simulink model "plotter_rigid_body"  (R2025a)
settings: Solver=VariableStepAuto  StartTime=0.0  StopTime=2  MaxStep=1e-3  RelTol=1e-3
values from neighbouring files (symbols this model uses):
  B_m = 0.000002    (= 2e-06)    [parameters.m]
  g = 9.8    [parameters.m]
  Gr = 1/30    (= 0.0333333333333)    [parameters.m]
  J_m = 0.000004    (= 4e-06)    [parameters.m]
  K_t = 0.009    [parameters.m]
  L = 0.3    [cinematic_sim.m]    (also in parameters.m)
  L_a = 0.0023    [parameters.m]
  m = 0.1    [parameters.m]
  R = 0.017    [parameters.m]
  R_a = 2.182    [parameters.m]
libraries: slpidlib x2
settings Model: SimulationMode=accelerator  Creator=bruno  LastModifiedBy=bruno

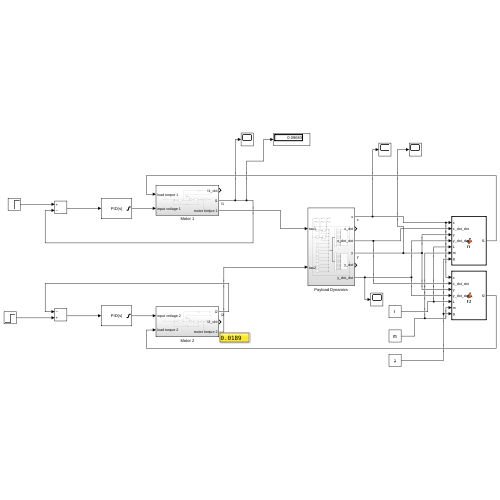
[thumbnail: Simulink's stored preview of the top-level diagram]
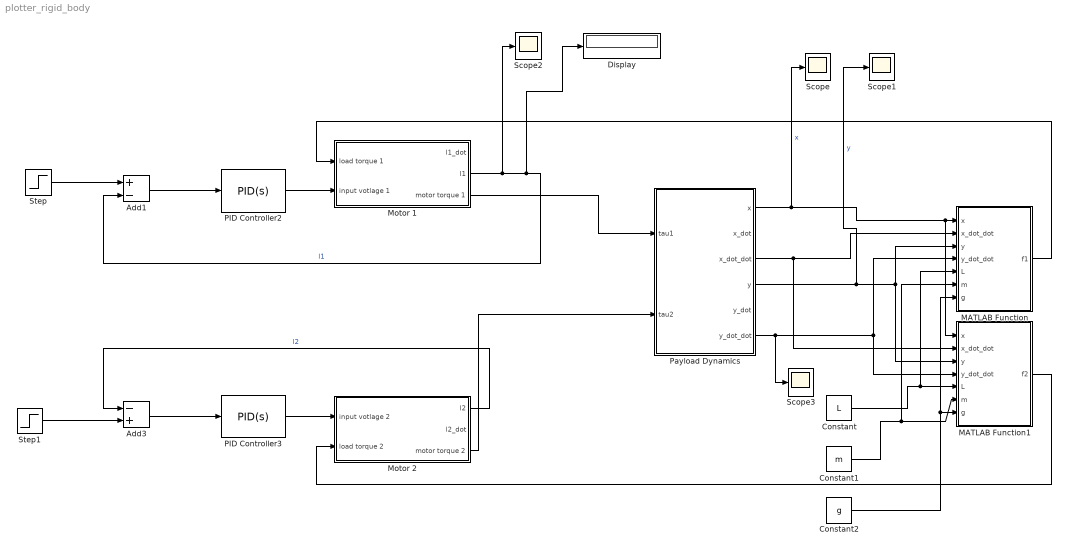
== system plotter_rigid_body ==
  Add1 : Sum  Inputs=+-
  Add3 : Sum  Inputs=-+
  Constant : Constant  Value=L
  Constant1 : Constant  Value=m
  Constant2 : Constant  Value=g
  Display : Display
  MATLAB Function : MATLAB Function  TreatAsAtomicUnit=on
  MATLAB Function1 : MATLAB Function  TreatAsAtomicUnit=on
  Motor 1 : Subsystem
  Motor 2 : Subsystem
  PID Controller2 : slpidlib/PID Controller  Controller=PID  Form=Parallel  TimeDomain=Continuous-time  UseExternalTs=off  SampleTime=-1  IntegratorMethod=Forward Euler  FilterMethod=Forward Euler  ControllerParametersSource=internal  P=7486.4932520919  I=24098.7164203864  UseKiTs=off  D=516.754104749892  UseExternalDerivativeSource=off  N=63057.2759663465  UseFilter=on  TunerSelectOption=Transfer Function Based (PID Tuner App)  InitialConditionSource=internal  InitialConditionForIntegrator=0  InitialConditionForFilter=0  DifferentiatorICPrevScaledInput=0  ExternalReset=none  TrackingMode=off  Kt=1  LimitOutput=on  SatLimitsSource=internal  UpperSaturationLimit=6  LowerSaturationLimit=-6  LinearizeAsGain=on  AntiWindupMode=none  Kb=1  LimitIntegrator=off  UpperIntegratorSaturationLimit=inf  LowerIntegratorSaturationLimit=-inf  POutMin=[]  POutMax=[]  IOutMin=[]  IOutMax=[]  DOutMin=[]  DOutMax=[]  NOutMin=[]  NOutMax=[]  SumOutMin=[]  SumOutMax=[]  SaturationOutMin=[]  SaturationOutMax=[]  PParamMin=[]  PParamMax=[]  IParamMin=[]  IParamMax=[]  DParamMin=[]  DParamMax=[]  NParamMin=[]  NParamMax=[]  KbParamMin=[]  KbParamMax=[]  KtParamMin=[]  KtParamMax=[]  KbOutMin=[]  KbOutMax=[]  KtOutMin=[]  KtOutMax=[]  IntegratorOutMin=[]  IntegratorOutMax=[]  FilterOutMin=[]  FilterOutMax=[]  SumI1OutMin=[]  SumI1OutMax=[]  SumI2OutMin=[]  SumI2OutMax=[]  SumI3OutMin=[]  SumI3OutMax=[]  SumI4OutMin=[]  SumI4OutMax=[]  SumDOutMin=[]  SumDOutMax=[]  DifferentiatorOutMin=[]  DifferentiatorOutMax=[]  FilterDiffOutCoefMin=[]  FilterDiffOutCoefMax=[]  ReciprocalOutMin=[]  ReciprocalOutMax=[]  SumDenOutMin=[]  SumDenOutMax=[]  SumNumOutMin=[]  SumNumOutMax=[]  DivideOutMin=[]  DivideOutMax=[]  UdiffTsProdOutMin=[]  UdiffTsProdOutMax=[]  NTsProdOutMin=[]  NTsProdOutMax=[]  UintegralTsProdOutMin=[]  UintegralTsProdOutMax=[]  UngainTsProdOutMin=[]  UngainTsProdOutMax=[]  ClampingZeroOutDataTypeStr=Inherit: Inherit via back propagation  ClampingZeroOutMin=[]  ClampingZeroOutMax=[]  FilterDenConstantOutDataTypeStr=Inherit: Inherit via back propagation  FilterDenConstantOutMin=[]  FilterDenConstantOutMax=[]  PCopyOutDataTypeStr=Inherit: Inherit via back propagation  PCopyOutMin=[]  PCopyOutMax=[]  NCopyOutDataTypeStr=Inherit: Inherit via back propagation  NCopyOutMin=[]  NCopyOutMax=[]  IntegratorContinuousStateAttributes=''  IntegratorStateMustResolveToSignalObject=off  IntegratorRTWStateStorageClass=Auto  FilterContinuousStateAttributes=''  FilterStateMustResolveToSignalObject=off  FilterRTWStateStorageClass=Auto  ParallelPVariant=InternalParameters  IdealPVariant=Disabled  IVariant=InternalParameters  DVariant=InternalParameters  IntegratorVariant=Continuous  SatVariant=Enabled  AWVariant=Passthrough  PCopyVariant=Disabled  TRVariant=Disabled  FdbkBlocksVariant=Forward  IdealPFdbkVariant=Disabled  SatFdbkVariant=Disabled  DerivativeFilterVariant=ContFilter  NVariant=InternalParameters  NCopyVariant=Disabled  FilterICVariant=InternalICsFilter  IntegratorICVariant=InternalICs  ExternalResetVariant=Disabled  TRSumVariant=Passthrough  SumFdbkVariant=Disabled  SumVariant=Sum_PID  TsampFilterVariant=InternalTs  TsampNgainVariant=Passthrough  TsampIntegralVariant=Disabled_SignalSpec  ExternalSaturationOutDataTypeStr=Inherit: Same as second input  DerivativeSourceVariant=ErrorSignal  PreIntVariant=InternalPreInt
  PID Controller3 : slpidlib/PID Controller  Controller=PID  Form=Parallel  TimeDomain=Continuous-time  UseExternalTs=off  SampleTime=-1  IntegratorMethod=Forward Euler  FilterMethod=Forward Euler  ControllerParametersSource=internal  P=7486.4932520919  I=24098.7164203864  UseKiTs=off  D=516.754104749892  UseExternalDerivativeSource=off  N=63057.2759663465  UseFilter=on  TunerSelectOption=Transfer Function Based (PID Tuner App)  InitialConditionSource=internal  InitialConditionForIntegrator=0  InitialConditionForFilter=0  DifferentiatorICPrevScaledInput=0  ExternalReset=none  TrackingMode=off  Kt=1  LimitOutput=on  SatLimitsSource=internal  UpperSaturationLimit=6  LowerSaturationLimit=-6  LinearizeAsGain=on  AntiWindupMode=none  Kb=1  LimitIntegrator=off  UpperIntegratorSaturationLimit=inf  LowerIntegratorSaturationLimit=-inf  POutMin=[]  POutMax=[]  IOutMin=[]  IOutMax=[]  DOutMin=[]  DOutMax=[]  NOutMin=[]  NOutMax=[]  SumOutMin=[]  SumOutMax=[]  SaturationOutMin=[]  SaturationOutMax=[]  PParamMin=[]  PParamMax=[]  IParamMin=[]  IParamMax=[]  DParamMin=[]  DParamMax=[]  NParamMin=[]  NParamMax=[]  KbParamMin=[]  KbParamMax=[]  KtParamMin=[]  KtParamMax=[]  KbOutMin=[]  KbOutMax=[]  KtOutMin=[]  KtOutMax=[]  IntegratorOutMin=[]  IntegratorOutMax=[]  FilterOutMin=[]  FilterOutMax=[]  SumI1OutMin=[]  SumI1OutMax=[]  SumI2OutMin=[]  SumI2OutMax=[]  SumI3OutMin=[]  SumI3OutMax=[]  SumI4OutMin=[]  SumI4OutMax=[]  SumDOutMin=[]  SumDOutMax=[]  DifferentiatorOutMin=[]  DifferentiatorOutMax=[]  FilterDiffOutCoefMin=[]  FilterDiffOutCoefMax=[]  ReciprocalOutMin=[]  ReciprocalOutMax=[]  SumDenOutMin=[]  SumDenOutMax=[]  SumNumOutMin=[]  SumNumOutMax=[]  DivideOutMin=[]  DivideOutMax=[]  UdiffTsProdOutMin=[]  UdiffTsProdOutMax=[]  NTsProdOutMin=[]  NTsProdOutMax=[]  UintegralTsProdOutMin=[]  UintegralTsProdOutMax=[]  UngainTsProdOutMin=[]  UngainTsProdOutMax=[]  ClampingZeroOutDataTypeStr=Inherit: Inherit via back propagation  ClampingZeroOutMin=[]  ClampingZeroOutMax=[]  FilterDenConstantOutDataTypeStr=Inherit: Inherit via back propagation  FilterDenConstantOutMin=[]  FilterDenConstantOutMax=[]  PCopyOutDataTypeStr=Inherit: Inherit via back propagation  PCopyOutMin=[]  PCopyOutMax=[]  NCopyOutDataTypeStr=Inherit: Inherit via back propagation  NCopyOutMin=[]  NCopyOutMax=[]  IntegratorContinuousStateAttributes=''  IntegratorStateMustResolveToSignalObject=off  IntegratorRTWStateStorageClass=Auto  FilterContinuousStateAttributes=''  FilterStateMustResolveToSignalObject=off  FilterRTWStateStorageClass=Auto  ParallelPVariant=InternalParameters  IdealPVariant=Disabled  IVariant=InternalParameters  DVariant=InternalParameters  IntegratorVariant=Continuous  SatVariant=Enabled  AWVariant=Passthrough  PCopyVariant=Disabled  TRVariant=Disabled  FdbkBlocksVariant=Forward  IdealPFdbkVariant=Disabled  SatFdbkVariant=Disabled  DerivativeFilterVariant=ContFilter  NVariant=InternalParameters  NCopyVariant=Disabled  FilterICVariant=InternalICsFilter  IntegratorICVariant=InternalICs  ExternalResetVariant=Disabled  TRSumVariant=Passthrough  SumFdbkVariant=Disabled  SumVariant=Sum_PID  TsampFilterVariant=InternalTs  TsampNgainVariant=Passthrough  TsampIntegralVariant=Disabled_SignalSpec  ExternalSaturationOutDataTypeStr=Inherit: Same as second input  DerivativeSourceVariant=ErrorSignal  PreIntVariant=InternalPreInt
  Payload Dynamics : Subsystem
  Scope{,1..3} (4 alike) : Scope
      Scope settings: ActiveDisplayYMinimum=0.1206169656337359  ActiveDisplayYMaximum=0.27436852673253087
      Scope1 settings: ActiveDisplayYMinimum=-0.00020832759673911072  ActiveDisplayYMaximum=0.18372931257695557
      Scope2 settings: ActiveDisplayYMinimum=-1  ActiveDisplayYMaximum=1  DataLoggingVariableName=ScopeData2
      Scope3 settings: ActiveDisplayYMinimum=-22.86647819571678  ActiveDisplayYMaximum=32.004217087156384  DataLoggingVariableName=ScopeData3
  Step : Step  Time=0  After=0.15  SampleTime=0
  Step1 : Step  Time=0  After=0.15  SampleTime=0
  wires:
  PID Controller2/1 -> Motor 1/2(input votlage 1)
  Add1/1 -> PID Controller2/1
  Step/1 -> Add1/1
  Add3/1 -> PID Controller3/1
  Step1/1 -> Add3/2
  Motor 1/2(l1) -> Scope2/1, Display/1, Add1/2  "l1"
  PID Controller3/1 -> Motor 2/1(input votlage 2)
  Motor 2/1(l2) -> Add3/1  "l2"
  Constant2/1 -> MATLAB Function1/7(g), MATLAB Function/7(g)
  Motor 2/3(motor torque 2) -> Payload Dynamics/2(tau2)
  Motor 1/3(motor torque 1) -> Payload Dynamics/1(tau1)
  Payload Dynamics/1(x) -> Scope/1, MATLAB Function1/1(x), MATLAB Function/1(x)  "x"
  Payload Dynamics/3(x_dot_dot) -> MATLAB Function1/2(x_dot_dot), MATLAB Function/2(x_dot_dot)
  Payload Dynamics/4(y) -> Scope1/1, MATLAB Function1/3(y), MATLAB Function/3(y)  "y"
  Payload Dynamics/6(y_dot_dot) -> Scope3/1, MATLAB Function1/4(y_dot_dot), MATLAB Function/4(y_dot_dot)
  Constant/1 -> MATLAB Function1/5(L), MATLAB Function/5(L)
  Constant1/1 -> MATLAB Function/6(m), MATLAB Function1/6(m)
  MATLAB Function/1(f1) -> Motor 1/1(load torque 1)
  MATLAB Function1/1(f2) -> Motor 2/2(load torque 2)

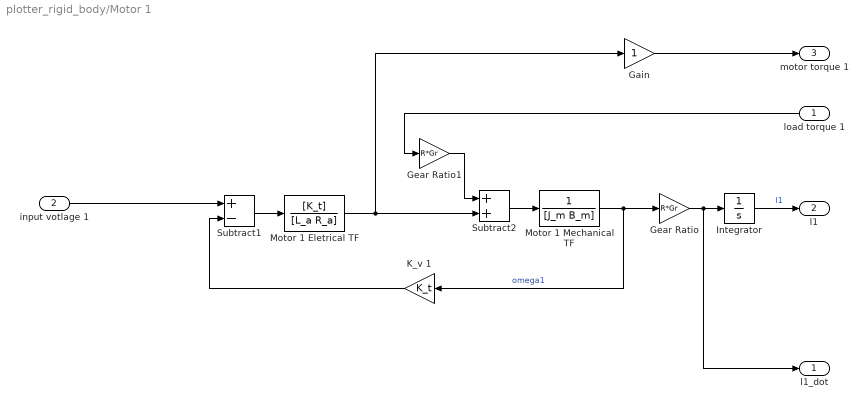
== system plotter_rigid_body/Motor 1 ==
  load torque 1 : Inport
  input votlage 1 : Inport  Port=2
  Gain : Gain
  Gear Ratio : Gain  Gain=R*Gr
  Gear Ratio1 : Gain  Gain=R*Gr
  Integrator : Integrator  InitialCondition=0.25
  K_v 1 : Gain  Gain=K_t
  Motor 1 Eletrical TF : TransferFcn  Numerator=[K_t]  Denominator=[L_a R_a]
  Motor 1 Mechanical TF : TransferFcn  Denominator=[J_m B_m]
  Subtract1 : Sum  Inputs=+-
  Subtract2 : Sum
  l1_dot : Outport
  l1 : Outport  Port=2
  motor torque 1 : Outport  Port=3
  wires:
  Motor 1 Eletrical TF/1 -> Gain/1, Subtract2/2
  load torque 1/1 -> Gear Ratio1/1
  K_v 1/1 -> Subtract1/2
  Gear Ratio1/1 -> Subtract2/1
  Subtract1/1 -> Motor 1 Eletrical TF/1
  Subtract2/1 -> Motor 1 Mechanical TF/1
  input votlage 1/1 -> Subtract1/1
  Motor 1 Mechanical TF/1 -> Gear Ratio/1, K_v 1/1  "omega1"
  Gear Ratio/1 -> l1_dot/1, Integrator/1
  Integrator/1 -> l1/1  "l1"
  Gain/1 -> motor torque 1/1

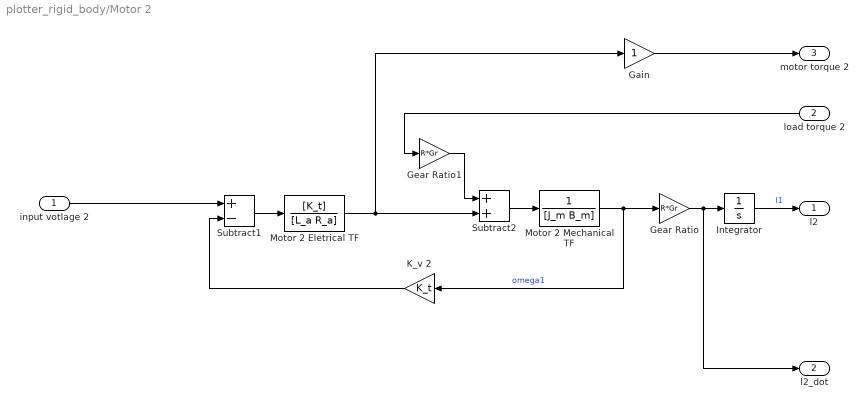
== system plotter_rigid_body/Motor 2 ==
  input votlage 2 : Inport
  load torque 2 : Inport  Port=2
  Gain : Gain
  Gear Ratio : Gain  Gain=R*Gr
  Gear Ratio1 : Gain  Gain=R*Gr
  Integrator : Integrator  InitialCondition=0.25
  K_v 2 : Gain  Gain=K_t
  Motor 2 Eletrical TF : TransferFcn  Numerator=[K_t]  Denominator=[L_a R_a]
  Motor 2 Mechanical TF : TransferFcn  Denominator=[J_m B_m]
  Subtract1 : Sum  Inputs=+-
  Subtract2 : Sum
  l2 : Outport
  l2_dot : Outport  Port=2
  motor torque 2 : Outport  Port=3
  wires:
  Motor 2 Eletrical TF/1 -> Gain/1, Subtract2/2
  load torque 2/1 -> Gear Ratio1/1
  K_v 2/1 -> Subtract1/2
  Gear Ratio1/1 -> Subtract2/1
  Subtract1/1 -> Motor 2 Eletrical TF/1
  Subtract2/1 -> Motor 2 Mechanical TF/1
  input votlage 2/1 -> Subtract1/1
  Motor 2 Mechanical TF/1 -> Gear Ratio/1, K_v 2/1  "omega1"
  Gear Ratio/1 -> l2_dot/1, Integrator/1
  Integrator/1 -> l2/1  "l1"
  Gain/1 -> motor torque 2/1

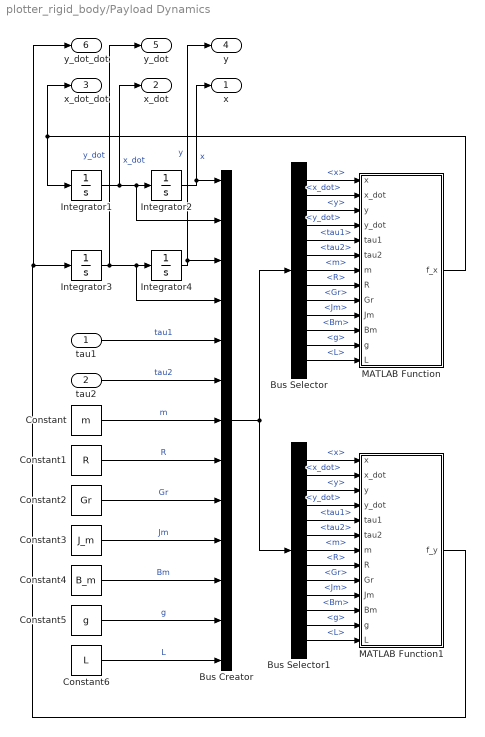
== system plotter_rigid_body/Payload Dynamics ==
  tau1 : Inport
  tau2 : Inport  Port=2
  Bus Creator : BusCreator  Inputs=13
  Bus Selector : BusSelector  OutputSignals=x,x_dot,y,y_dot,tau1,tau2,m,R,Gr,Jm,Bm,g,L
  Bus Selector1 : BusSelector  OutputSignals=x,x_dot,y,y_dot,tau1,tau2,m,R,Gr,Jm,Bm,g,L
  Constant : Constant  Value=m
  Constant1 : Constant  Value=R
  Constant2 : Constant  Value=Gr
  Constant3 : Constant  Value=J_m
  Constant4 : Constant  Value=B_m
  Constant5 : Constant  Value=g
  Constant6 : Constant  Value=L
  Integrator1 : Integrator
  Integrator2 : Integrator  InitialCondition=0.15
  Integrator3 : Integrator
  Integrator4 : Integrator  InitialCondition=0.2
  MATLAB Function : MATLAB Function  TreatAsAtomicUnit=on
  MATLAB Function1 : MATLAB Function  TreatAsAtomicUnit=on
  x : Outport
  x_dot : Outport  Port=2
  x_dot_dot : Outport  Port=3
  y : Outport  Port=4
  y_dot : Outport  Port=5
  y_dot_dot : Outport  Port=6
  wires:
  Integrator1/1 -> x_dot/1, Bus Creator/2, Integrator2/1  "x_dot"
  Integrator3/1 -> y_dot/1, Bus Creator/4, Integrator4/1  "y_dot"
  MATLAB Function/1(f_x) -> x_dot_dot/1, Integrator1/1
  MATLAB Function1/1(f_y) -> y_dot_dot/1, Integrator3/1
  Integrator2/1 -> x/1, Bus Creator/1  "x"
  Integrator4/1 -> y/1, Bus Creator/3  "y"
  tau1/1 -> Bus Creator/5  "tau1"
  tau2/1 -> Bus Creator/6  "tau2"
  Constant/1 -> Bus Creator/7  "m"
  Constant1/1 -> Bus Creator/8  "R"
  Constant2/1 -> Bus Creator/9  "Gr"
  Constant3/1 -> Bus Creator/10  "Jm"
  Constant4/1 -> Bus Creator/11  "Bm"
  Constant5/1 -> Bus Creator/12  "g"
  Bus Creator/1 -> Bus Selector/1, Bus Selector1/1
  Bus Selector/1 -> MATLAB Function/1(x)  "<x>"
  Bus Selector/2 -> MATLAB Function/2(x_dot)  "<x_dot>"
  Bus Selector/3 -> MATLAB Function/3(y)  "<y>"
  Bus Selector/4 -> MATLAB Function/4(y_dot)  "<y_dot>"
  Bus Selector/5 -> MATLAB Function/5(tau1)  "<tau1>"
  Bus Selector/6 -> MATLAB Function/6(tau2)  "<tau2>"
  Bus Selector/7 -> MATLAB Function/7(m)  "<m>"
  Bus Selector/8 -> MATLAB Function/8(R)  "<R>"
  Bus Selector/9 -> MATLAB Function/9(Gr)  "<Gr>"
  Bus Selector/10 -> MATLAB Function/10(Jm)  "<Jm>"
  Bus Selector/11 -> MATLAB Function/11(Bm)  "<Bm>"
  Bus Selector/12 -> MATLAB Function/12(g)  "<g>"
  Bus Selector1/1 -> MATLAB Function1/1(x)  "<x>"
  Bus Selector1/2 -> MATLAB Function1/2(x_dot)  "<x_dot>"
  Bus Selector1/3 -> MATLAB Function1/3(y)  "<y>"
  Bus Selector1/4 -> MATLAB Function1/4(y_dot)  "<y_dot>"
  Bus Selector1/5 -> MATLAB Function1/5(tau1)  "<tau1>"
  Bus Selector1/6 -> MATLAB Function1/6(tau2)  "<tau2>"
  Bus Selector1/7 -> MATLAB Function1/7(m)  "<m>"
  Bus Selector1/8 -> MATLAB Function1/8(R)  "<R>"
  Bus Selector1/9 -> MATLAB Function1/9(Gr)  "<Gr>"
  Bus Selector1/10 -> MATLAB Function1/10(Jm)  "<Jm>"
  Bus Selector1/11 -> MATLAB Function1/11(Bm)  "<Bm>"
  Bus Selector1/12 -> MATLAB Function1/12(g)  "<g>"
  Constant6/1 -> Bus Creator/13  "L"
  Bus Selector/13 -> MATLAB Function/13(L)  "<L>"
  Bus Selector1/13 -> MATLAB Function1/13(L)  "<L>"

== matlab function plotter_rigid_body/Payload Dynamics/MATLAB Function1 ==
  data: x input; f_y output; x_dot input; y input; y_dot input; tau1 input; tau2 input; m input; R input; Gr input; Jm input; Bm input; g input; L input
function f_y = f_y(x,x_dot,y,y_dot,tau1, tau2, m,R,Gr,Jm,Bm,g,L)
    a11 = m + Jm/(R*Gr)^2*(x^2/(x^2 + y^2) + (L-x)^2/((L-x)^2+y^2));
    a12 = Jm/(R*Gr)^2*(x*y/(x^2 + y^2) - (L-x)*y/((L-x)^2+y^2));
    a21 = a12;
    a22 = m + Jm/(R*Gr)^2*(y^2/(x^2 + y^2) + y^2/((L-x)^2+y^2));
    b1 = -x/sqrt(x^2+y^2)*(Jm/(R*Gr)^2*((x_dot^2+y_dot^2)*sqrt(x^2+y^2)-(x*x_dot+y*y_dot)^2/sqrt(x^2+y^2))/(x^2+y^2)+Bm*(x*x_dot+y*y_dot)/((R*Gr)^2*sqrt(x^2+y^2))-tau1/(R*Gr)) ...
         + (L-x)/sqrt((L-x)^2+y^2)*(Jm/(R*Gr)^2*((x_dot^2+y_dot^2)*sqrt((L-x)^2+y^2)-(-(L-x)*x_dot+y*y_dot)^2/sqrt((L-x)^2+y^2))/((L-x)^2+y^2)+Bm*(-(L-x)*x_dot+y*y_dot)/((R*Gr)^2*sqrt((L-x)^2+y^2))-tau2/(R*Gr));
    b2 = m*g -y/sqrt(x^2+y^2)*(Jm/(R*Gr)^2*((x_dot^2+y_dot^2)*sqrt(x^2+y^2)-(x*x_dot+y*y_dot)^2/sqrt(x^2+y^2))/(x^2+y^2)+Bm*(x*x_dot+y*y_dot)/((R*Gr)^2*sqrt(x^2+y^2))-tau1/(R*Gr)) ...
         -y/sqrt((L-x)^2+y^2)*(Jm/(R*Gr)^2*((x_dot^2+y_dot^2)*sqrt((L-x)^2+y^2)-(-(L-x)*x_dot+y*y_dot)^2/sqrt((L-x)^2+y^2))/((L-x)^2+y^2)+Bm*(-(L-x)*x_dot+y*y_dot)/((R*Gr)^2*sqrt((L-x)^2+y^2))-tau2/(R*Gr));
    f_y = (b2 -a21/a11*b1)/(a22-a21*a12/a11);

== matlab function plotter_rigid_body/Payload Dynamics/MATLAB Function ==
  data: x input; f_x output; x_dot input; y input; y_dot input; tau1 input; tau2 input; m input; R input; Gr input; Jm input; Bm input; g input; L input
function f_x = f_x(x,x_dot,y,y_dot,tau1, tau2, m,R,Gr,Jm,Bm,g,L)
    a11 = m + Jm/(R*Gr)^2*(x^2/(x^2 + y^2) + (L-x)^2/((L-x)^2+y^2));
    a12 = Jm/(R*Gr)^2*(x*y/(x^2 + y^2) - (L-x)*y/((L-x)^2+y^2));
    a21 = a12;
    a22 = m + Jm/(R*Gr)^2*(y^2/(x^2 + y^2) + y^2/((L-x)^2+y^2));
    b1 = -x/sqrt(x^2+y^2)*(Jm/(R*Gr)^2*((x_dot^2+y_dot^2)*sqrt(x^2+y^2)-(x*x_dot+y*y_dot)^2/sqrt(x^2+y^2))/(x^2+y^2)+Bm*(x*x_dot+y*y_dot)/((R*Gr)^2*sqrt(x^2+y^2))-tau1/(R*Gr)) ...
         + (L-x)/sqrt((L-x)^2+y^2)*(Jm/(R*Gr)^2*((x_dot^2+y_dot^2)*sqrt((L-x)^2+y^2)-(-(L-x)*x_dot+y*y_dot)^2/sqrt((L-x)^2+y^2))/((L-x)^2+y^2)+Bm*(-(L-x)*x_dot+y*y_dot)/((R*Gr)^2*sqrt((L-x)^2+y^2))-tau2/(R*Gr));
    b2 = m*g -y/sqrt(x^2+y^2)*(Jm/(R*Gr)^2*((x_dot^2+y_dot^2)*sqrt(x^2+y^2)-(x*x_dot+y*y_dot)^2/sqrt(x^2+y^2))/(x^2+y^2)+Bm*(x*x_dot+y*y_dot)/((R*Gr)^2*sqrt(x^2+y^2))-tau1/(R*Gr)) ...
         -y/sqrt((L-x)^2+y^2)*(Jm/(R*Gr)^2*((x_dot^2+y_dot^2)*sqrt((L-x)^2+y^2)-(-(L-x)*x_dot+y*y_dot)^2/sqrt((L-x)^2+y^2))/((L-x)^2+y^2)+Bm*(-(L-x)*x_dot+y*y_dot)/((R*Gr)^2*sqrt((L-x)^2+y^2))-tau2/(R*Gr));
    f_x = (b1 - a12*(b2-a21/a11-b1)/(a22-a21*a12/a11))/a11

== matlab function plotter_rigid_body/MATLAB Function ==
  data: x input; f1 output; x_dot_dot input; y input; y_dot_dot input; L input; m input; g input
function f1 = f1(x,x_dot_dot,y,y_dot_dot,L,m,g)

f1 = m*sqrt(x^2+y^2)*(L-x)*(x_dot_dot*y/x+g-y_dot_dot)/((L-x)+y-x_dot_dot/x);

== matlab function plotter_rigid_body/MATLAB Function1 ==
  data: x input; f2 output; x_dot_dot input; y input; y_dot_dot input; L input; m input; g input
function f2 = f2(x,x_dot_dot,y,y_dot_dot,L,m,g)

f2 = m*sqrt((L-x)^2+y^2)*(x_dot_dot*y/x+g-y_dot_dot)/((L-x));
